simulink model "check_ndtm_varyingEnvironment"  (R2018b)
settings: configuration reference "Physics" (kept outside this file)
settings Model: DataDictionary=check_ndtm.sldd  OrderedModelArguments=off  Creator=wischnewski  LastModifiedBy=ga25xiw

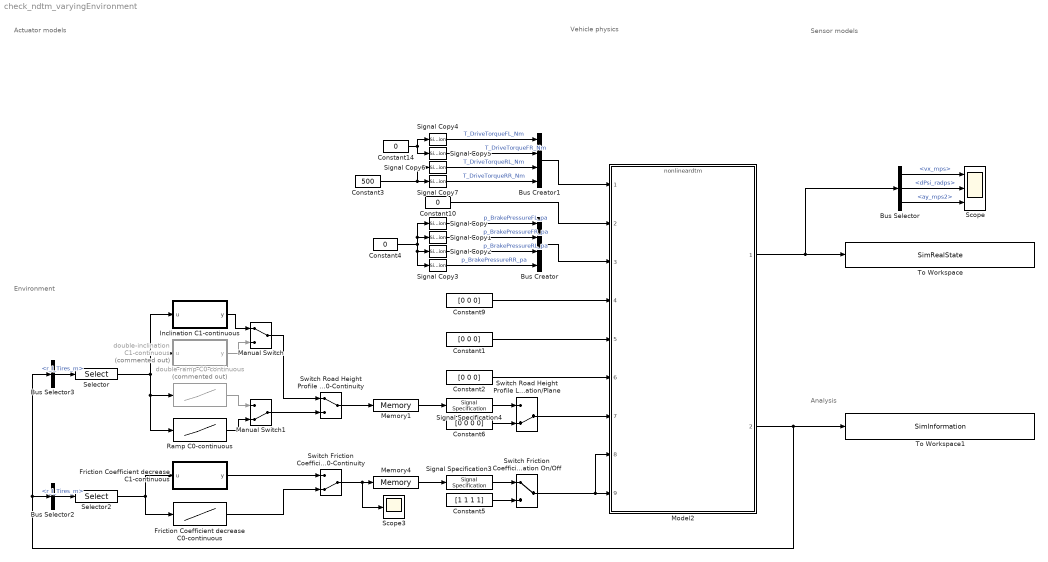
== system check_ndtm_varyingEnvironment ==
  note: Actuator models
  note: Vehicle physics
  note: Environment
  note: Analysis
  note: Sensor models
  Bus Creator : BusCreator  Inputs=4  OutDataTypeStr=Bus: BrakePressure_Pa
  Bus Creator1 : BusCreator  Inputs=4  OutDataTypeStr=Bus: DriveTorque_Nm
  Bus Selector : BusSelector  OutputSignals=vx_mps,dPsi_radps,ay_mps2
  Bus Selector2 : BusSelector  OutputSignals=Wheel.r_I_Tires_m
  Bus Selector3 : BusSelector  OutputSignals=Wheel.r_I_Tires_m
  Constant1 : Constant  Value=[0 0 0]
  Constant10 : Constant  Value=0
  Constant14 : Constant  Value=0
  Constant2 : Constant  Value=[0 0 0]
  Constant3 : Constant  Value=500
  Constant4 : Constant  Value=0
  Constant5 : Constant  Value=[1 1 1 1]
  Constant6 : Constant  Value=[0 0 0 0]
  Constant9 : Constant  Value=[0 0 0]
  Friction Coefficient decrease C0-continuous : Lookup_n-D  NumberOfTableDimensions=1  BreakpointsForDimension1=[0 250 350 500]  Table=[1 1 0.25 0.25]  InternalRulePriority=Speed  RndMeth=Simplest  InputSameDT=on
  Friction Coefficient decrease C1-continuous : MATLAB Function  TreatAsAtomicUnit=on
  Inclination C1-continuous : MATLAB Function  TreatAsAtomicUnit=on
  Manual Switch : ManualSwitch
  Manual Switch1 : ManualSwitch  CurrentSetting=0
  Memory1 : Memory
  Memory4 : Memory
  Model2 : ModelReference  ModelNameDialog=nonlineardtm  ParameterArgumentNames=x0_initialstates  ParameterArgumentValues=[0 0 0 0 0 -pi/2]  UsingDefaultArgumentValue=0  SimulationMode=Normal  ModelReferenceVersion=1.642
  Ramp C0-continuous : Lookup_n-D  NumberOfTableDimensions=1  BreakpointsForDimension1=[0 100 500 1000]  Table=[0 0 -20 -20]  InternalRulePriority=Speed  RndMeth=Simplest  InputSameDT=on
  Scope : Scope  NumInputPorts=3
  Scope3 : Scope
  Selector : Selector  NumberOfDimensions=2  InputPortWidth=3  IndexOptions=Index vector (dialog),Select all  Indices=1,1  OutputSizes=1,1
  Selector2 : Selector  NumberOfDimensions=2  InputPortWidth=3  IndexOptions=Index vector (dialog),Select all  Indices=1,1  OutputSizes=1,1
  Signal Copy{,1..7} (8 alike) : SignalConversion  OverrideOpt=off
  Signal Specification3 : SignalSpecification  Dimensions=[1 4]
  Signal Specification4 : SignalSpecification  Dimensions=[1 4]
  Switch Friction Coefficient Variation C1-Continuity/C0-Continuity : ManualSwitch  CurrentSetting=0
  Switch Friction Coefficient Variation On/Off : ManualSwitch
  Switch Road Height Profile C1-Continuity/C0-Continuity : ManualSwitch
  Switch Road Height Profile Longitudinal Inclination/Plane : ManualSwitch  CurrentSetting=0
  To Workspace : ToWorkspace  VariableName=SimRealState  SaveFormat=Timeseries  SampleTime=-1
  To Workspace1 : ToWorkspace  VariableName=SimInformation  SaveFormat=Timeseries  SampleTime=-1
  double-inclination C1-continuous : MATLAB Function  Commented=on  TreatAsAtomicUnit=on
  double-ramp-C0-continuous : Lookup_n-D  Commented=on  NumberOfTableDimensions=1  BreakpointsForDimension1=[0 100 500 700 1100 2000]  Table=[0 0 -20 -20 0 0]  InternalRulePriority=Speed  RndMeth=Simplest  InputSameDT=on
  wires:
  Bus Selector/1 -> Scope/1  "<vx_mps>"
  Bus Selector/2 -> Scope/2  "<dPsi_radps>"
  Bus Selector/3 -> Scope/3  "<ay_mps2>"
  Model2/1 -> Bus Selector/1, To Workspace/1
  Constant9/1 -> Model2/4
  Constant1/1 -> Model2/5
  Constant2/1 -> Model2/6
  Switch Friction Coefficient Variation On/Off/1 -> Model2/8, Model2/9
  Bus Selector3/1 -> Selector/1  "<r_I_Tires_m>"
  Constant6/1 -> Switch Road Height Profile Longitudinal Inclination/Plane/2
  Model2/2 -> To Workspace1/1, Bus Selector3/1, Bus Selector2/1
  Switch Road Height Profile Longitudinal Inclination/Plane/1 -> Model2/7
  Selector/1 -> double-ramp-C0-continuous/1, Ramp C0-continuous/1, double-inclination C1-continuous/1(u), Inclination C1-continuous/1(u)
  Switch Road Height Profile C1-Continuity/C0-Continuity/1 -> Memory1/1
  Ramp C0-continuous/1 -> Manual Switch1/2
  Inclination C1-continuous/1(y) -> Manual Switch/1
  Manual Switch1/1 -> Switch Road Height Profile C1-Continuity/C0-Continuity/2
  Manual Switch/1 -> Switch Road Height Profile C1-Continuity/C0-Continuity/1
  Bus Selector2/1 -> Selector2/1  "<r_I_Tires_m>"
  Selector2/1 -> Friction Coefficient decrease C0-continuous/1, Friction Coefficient decrease C1-continuous/1(u)
  Constant5/1 -> Switch Friction Coefficient Variation On/Off/2
  Switch Friction Coefficient Variation C1-Continuity/C0-Continuity/1 -> Scope3/1, Memory4/1
  Friction Coefficient decrease C0-continuous/1 -> Switch Friction Coefficient Variation C1-Continuity/C0-Continuity/2
  Friction Coefficient decrease C1-continuous/1(y) -> Switch Friction Coefficient Variation C1-Continuity/C0-Continuity/1
  Signal Specification3/1 -> Switch Friction Coefficient Variation On/Off/1
  Signal Specification4/1 -> Switch Road Height Profile Longitudinal Inclination/Plane/1
  double-inclination C1-continuous/1(y) -> Manual Switch/2
  double-ramp-C0-continuous/1 -> Manual Switch1/1
  Memory1/1 -> Signal Specification4/1
  Memory4/1 -> Signal Specification3/1
  Signal Copy2/1 -> Bus Creator/3  "p_BrakePressureRL_pa"
  Constant3/1 -> Signal Copy6/1, Signal Copy7/1
  Signal Copy/1 -> Bus Creator/1  "p_BrakePressureFL_pa"
  Signal Copy1/1 -> Bus Creator/2  "p_BrakePressureFR_pa"
  Bus Creator/1 -> Model2/3
  Constant10/1 -> Model2/2
  Bus Creator1/1 -> Model2/1
  Signal Copy5/1 -> Bus Creator1/2  "T_DriveTorqueFR_Nm"
  Signal Copy7/1 -> Bus Creator1/4  "T_DriveTorqueRR_Nm"
  Signal Copy4/1 -> Bus Creator1/1  "T_DriveTorqueFL_Nm"
  Signal Copy6/1 -> Bus Creator1/3  "T_DriveTorqueRL_Nm"
  Signal Copy3/1 -> Bus Creator/4  "p_BrakePressureRR_pa"
  Constant14/1 -> Signal Copy4/1, Signal Copy5/1
  Constant4/1 -> Signal Copy/1, Signal Copy1/1, Signal Copy3/1, Signal Copy2/1

== matlab function check_ndtm_varyingEnvironment/Inclination C1-continuous ==
  data: u input; y output
function y = fcn(u)

profil=zeros(1,4);

for i=1:4

if u(i)<=100
    profil(i)=0;
elseif u(i)>100 && u(i)<500
    profil(i)=-10-10*sin(pi/400*(u(i)-300));
elseif u(i)>=500
    profil(i)=-20;    
end    

y=profil;

end

== matlab function check_ndtm_varyingEnvironment/double-inclination C1-continuous ==
  data: u input; y output
function y = fcn(u)

profil=zeros(1,4);

for i=1:4
    
if u(i)>100 && u(i)<500
    profil(i)=-10-10*sin(pi/400*(u(i)-300));
elseif u(i)>=500 && u(i)<=700
    profil(i)=-20;
elseif u(i)>700 && u(i)<1100
    profil(i)=-10+10*sin(pi/400*(u(i)-900));
else
    profil(i)=0;
    
end    

y=profil;

end

== matlab function check_ndtm_varyingEnvironment/Friction Coefficient decrease C1-continuous ==
  data: u input; y output
function y = fcn(u)

reibung=zeros(1,4);

for i=1:4

if u(i)<=500
    reibung(i)=1;
elseif u(i)>500 && u(i)<750
    reibung(i)=1.25/2-0.75/2*sin(pi/250*(u(i)-625));
elseif u(i)>=500
    reibung(i)=0.25;    
end    

y=reibung;

end
